simulink model "normalization"  (R2024a)
settings: Solver=VariableStepAuto  StartTime=0.0  StopTime=20  RelTol=1e-3
InitFcn:
  | COL=256;
  | ROW=384;
  | NUM=6;
  | K_COL=COL;
  | K_ROW=ROW/NUM;
  | PLIO_NUM=3;
  | 
  | mtxA_w = [];
  | for i=0:2
  |     pattern = struct('buffer_dimension', [COL,ROW], 'tiling_dimension', [COL,ROW/PLIO_NUM], 'offset', [0,ROW/PLIO_NUM*i]);
  |     mtxA_w = [mtxA_w, pattern];
  | end
  | 
  | mtxA_r = [];
  | for i=0:5
  |     pattern = struct('buffer_dimension', [COL,ROW], 'tiling_dimension', [K_COL,K_ROW], 'offset', [0,K_ROW*i]);
  |     mtxA_r = [mtxA_r, pattern];
  | end
  | 
  | mtxB_w = [];
  | for i=0:5
  |     pattern = struct('buffer_dimension', [COL,ROW], 'tiling_dimension', [K_COL,K_ROW], 'offset', [0,K_ROW*i]);
  |     mtxB_w = [mtxB_w, pattern];
  | end
  | 
  | mtxB_r = [];
  | for i=0:2
  |     pattern = struct('buffer_dimension', [COL,ROW], 'tiling_dimension', [COL,ROW/PLIO_NUM], 'offset', [0,ROW/PLIO_NUM*i]);
  |     mtxB_r = [mtxB_r, pattern];
  | end
  | 
  | inMat = randn(ROW,COL,'single')*2^14;
  | inMatNormalized= (inMat-mean(inMat,'all'))/std(inMat,1,'all');
undefined symbols (not defined in the file or in its folder): aie, AIE, mean_dev_norm_first, mean_dev_norm_last, mean_dev_norm_middle, ML, S, vsvh1760, xcve2802
libraries: aieBasic x14, aieUtilities x10, dspstat3 x2, vmcUtilities x1
settings Model: Creator=robg  LastModifiedBy=sdegala
settings DataIOCC: ReturnWorkspaceOutputs=off
settings SFSimCC: SimTargetLang=C++
settings RTWCC: GPUComputeCapability=3.5

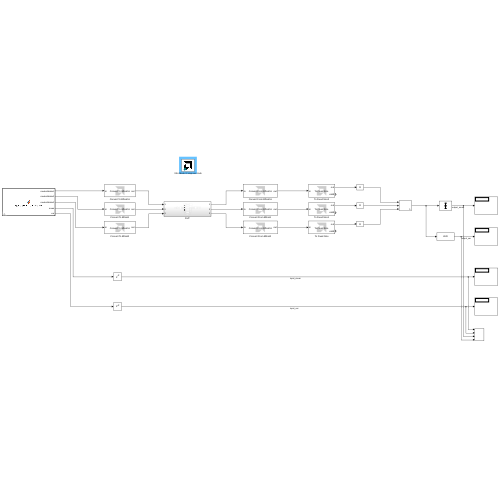
[thumbnail: Simulink's stored preview of the top-level diagram]
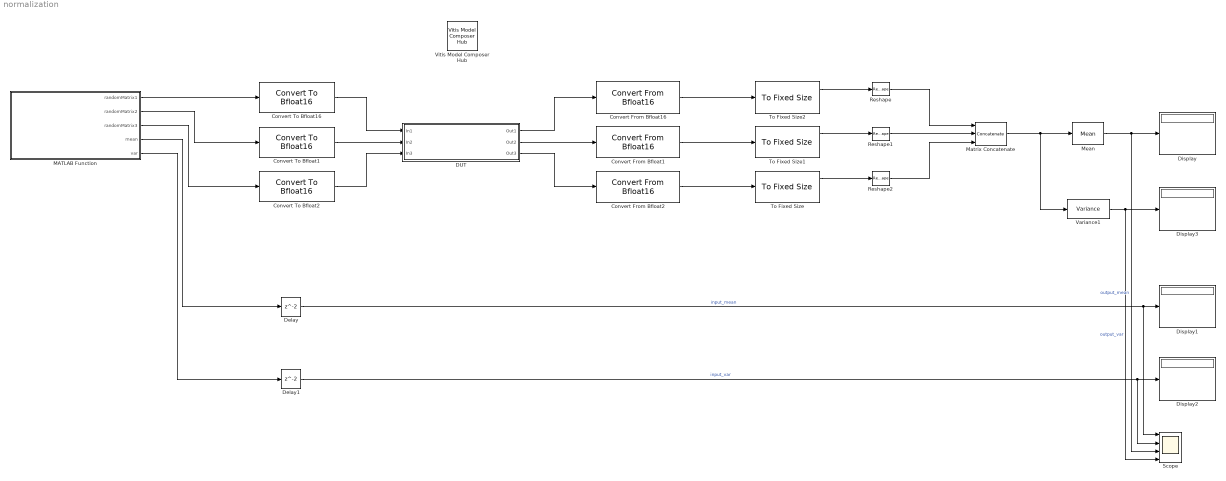
== system normalization ==
  Convert From Bfloat1 : aieUtilities/Convert From Bfloat16  OutputDataType=single
  Convert From Bfloat16 : aieUtilities/Convert From Bfloat16  OutputDataType=single
  Convert From Bfloat2 : aieUtilities/Convert From Bfloat16  OutputDataType=single
  Convert To Bfloat1 : aieUtilities/Convert To Bfloat16
  Convert To Bfloat16 : aieUtilities/Convert To Bfloat16
  Convert To Bfloat2 : aieUtilities/Convert To Bfloat16
  DUT : Subsystem
  Delay : Delay
  Delay1 : Delay
  Display{,1..3} (4 alike) : Display
  MATLAB Function : MATLAB Function  TreatAsAtomicUnit=on  mask{numRows=ROW, numCols=COL}
      mask prompts: numRows "Number of Rows"; numCols "Number of  Columns"
  Matrix Concatenate : Concatenate  NumInputs=3  Mode=Multidimensional array
  Mean : dspstat3/Mean  run=off  InputProcessing=Columns as channels (frame based)  reset_popup=None  directionMode=Entire input  dimension=1  roiEnable=off  roiType=Rectangles  roiPortion=Entire ROI  roiOutput=Individual statistics for each ROI  roiFlag=off  roundingMode=Floor  overflowMode=off  outputDataTypeStr=Inherit: Same as accumulator  outputMin=[]  outputMax=[]  outputLastDataTypeStr=Inherit: Same as accumulator
  Reshape : Reshape  OutputDimensionality=Customize  OutputDimensions=[ROW/PLIO_NUM,COL]
  Reshape1 : Reshape  OutputDimensionality=Customize  OutputDimensions=[ROW/PLIO_NUM,COL]
  Reshape2 : Reshape  OutputDimensionality=Customize  OutputDimensions=[ROW/PLIO_NUM,COL]
  Scope : Scope  NumInputPorts=4
  To Fixed Size : aieUtilities/To Fixed Size  Mode=Produce a valid output signal  OutputSize=Inherit: Same as input  CopyMethod=Buffer samples to form output  HasStatusOutput=on
  To Fixed Size1 : aieUtilities/To Fixed Size  Mode=Produce a valid output signal  OutputSize=Inherit: Same as input  CopyMethod=Buffer samples to form output  HasStatusOutput=on
  To Fixed Size2 : aieUtilities/To Fixed Size  Mode=Produce a valid output signal  OutputSize=Inherit: Same as input  CopyMethod=Buffer samples to form output  HasStatusOutput=on
  Variance1 : dspstat3/Variance  run=off  InputProcessing=Columns as channels (frame based)  reset_popup=None  directionMode=Entire input  dimension=1  roiEnable=off  roiType=Rectangles  roiPortion=Entire ROI  roiOutput=Individual statistics for each ROI  roiFlag=off  roundingMode=Floor  overflowMode=off
  Vitis Model Composer Hub : vmcUtilities/Vitis Model Composer Hub  Tag=genX  CodeGeneration=off  SubsystemName=DUT  BlockHierPath=normalization/DUT  CompilationType=HWCompilation  SubsystemType=AIENode  ExportTypeV2=Graph Code  AIEArrayConfig=Use entire AIE array  StartColumn=1  NumberOfColumns=1  TargetDirectory=./code  exportDesign=on  analyzeDesign=off  validateDesignOnHw=off  ExportType=HW Code  IpVendor=xilinx.com  IpLibrary=hls  IpVersion=1.0  IpHWLanguage=Verilog  AieCompilerOptions={}  AieSimulatorOptions={}  CreateTestbench=off  TestbenchStackSize=10  RunRtlSim=off  RunCSim=off  RunAieSim=on  AieSimTimeout=50000  RunAieSimProfiling=off  LaunchVitisAnalyzer=off  PlotOutput=off  RunX86Sim=off  X86SimTimeout=10  GenHwImage=off  GenLibadfXo=off  GenHwValidationCode=off  PlatformType=Not Specified  HwSystemType=Baremetal  HwValidationTarget=hw  ProjDevice=xcve2802-vsvh1760-2MP-e-S  ProjDevicePart=xcve2802-vsvh1760-2MP-e-S  AIEType=AIE-ML  SamplePeriod=-1  ClockFrequency=200  DataPathParallelism=1  xilinxfamily=versalaiedge  part=xcve2802  speed=-2MP-e-S  package=vsvh1760  directory=./netlist  testbench=off  incr_netlist=off  synthesis_tool=Vivado  clock_wrapper=Clock Enables  dbl_ovrd=According to Block Masks  dcm_input_clock_period=10  sysclk_period=10  simulink_period=1  eval_field=0  IPInfoJsonString="{\"DUTSubsystemName\":\"DUT\",\"AIESubsystem\":{\"SubsystemName\":\"DUT\",\"TargetDirectory\":\"./code\",\"AIEArrayConfig\":\"Use entire AIE array\",\"StartColumn\":\"0\",\"NumberOfColumns\":\"1\"},\"SubsystemTag\":\"AIENode\"}"  LogFileName=/proj/xhdhdstaff5/sdegala/Head1/HEAD/VMC_2025_2_July/Examples/AIENGINE/Normalization/code/model_composer.log  NThreads=4  IPConfigFile=/tmp/vmctmp-6835010160091439353/normalization_ipconfig.json
  wires:
  DUT/1(Out1) -> Convert From Bfloat16/1
  DUT/2(Out2) -> Convert From Bfloat1/1
  DUT/3(Out3) -> Convert From Bfloat2/1
  Convert From Bfloat16/1 -> To Fixed Size2/1
  Convert From Bfloat1/1 -> To Fixed Size1/1
  Convert From Bfloat2/1 -> To Fixed Size/1
  To Fixed Size2/1 -> Reshape/1
  To Fixed Size1/1 -> Reshape1/1
  To Fixed Size/1 -> Reshape2/1
  Reshape/1 -> Matrix Concatenate/1
  Reshape1/1 -> Matrix Concatenate/2
  Reshape2/1 -> Matrix Concatenate/3
  Matrix Concatenate/1 -> Variance1/1, Mean/1
  Mean/1 -> Scope/3, Display/1  "output_mean"
  MATLAB Function/5(var) -> Delay1/1
  Variance1/1 -> Scope/4, Display3/1  "output_var"
  MATLAB Function/4(mean) -> Delay/1
  MATLAB Function/1(randomMatrix1) -> Convert To Bfloat16/1
  MATLAB Function/2(randomMatrix2) -> Convert To Bfloat1/1
  MATLAB Function/3(randomMatrix3) -> Convert To Bfloat2/1
  Convert To Bfloat16/1 -> DUT/1(In1)
  Convert To Bfloat1/1 -> DUT/2(In2)
  Convert To Bfloat2/1 -> DUT/3(In3)
  Delay/1 -> Scope/1, Display1/1  "input_mean"
  Delay1/1 -> Scope/2, Display2/1  "input_var"

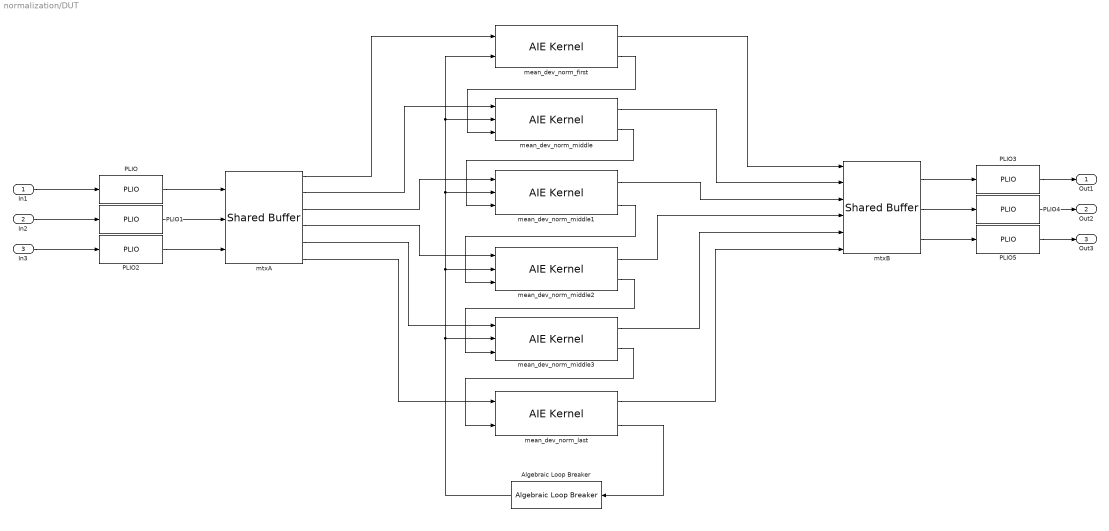
== system normalization/DUT ==
  In1 : Inport
  In2 : Inport  Port=2
  In3 : Inport  Port=3
  Algebraic Loop Breaker : aieUtilities/Algebraic Loop Breaker
  PLIO{,1..5} (6 alike) : aieBasic/PLIO  PlioWidth=128  PlioFreqSpec=off  PlioFreq=250  ColLocation=0  channel=0  blockJsonConstraints=[]  deprecateConstraints=0
  mean_dev_norm_first : aieBasic/AIE Kernel  KernelAllAttrs=|  PortNames={'data'; 'mean_dev'; 'out'; 'partial_out'}  PortSerializedTypes={'{Q2{R{Tadf::input_buffer{1{t{Sbfloat16}}}}}}'; '{Q2{P{Tinput_stream{1{t{Sbfloat16}}}}}}'; '{Q2{R{Tadf::output_buffer{1{t{Sbfloat16}}}}}}'; '{Q2{P{Toutput_cascade{2{t{Saccfloat}}{t{Bv}}}}}}'}  PortWindowSizes={1.600000000000000000e+01, 0.000000000000000000e+00, 1.600000000000000000e+01, 0.000000000000000000e+00}  PortWindowMargins={0.000000000000000000e+00, 0.000000000000000000e+00, 0.000000000000000000e+00, 0.000000000000000000e+00}  PortSynchronicities={'sync', 'auto', 'sync', 'auto'}  PortSignalSizes={0.000000000000000000e+00; 0.000000000000000000e+00; 0.000000000000000000e+00; 3.200000000000000000e+01}  FunctionTemplateSpecKind=implicit  FunctionTemplateParamNames={'COL'; 'ROW'}  FunctionTemplateParamKinds={'nontype'; 'nontype'}  FunctionTemplateParamTypes={'int'; 'int'}  FunctionTemplateParamValues={'0', '0'}  FunctionIndex=1  FunctionTabVisible=on  FunctionTemplateParamsVisible=on  FunctionDeclTypeOptions=|  FunctionDecl=|  FunctionTemplateParams={ 'COL', 'int', 'K_COL'; 'ROW', 'int', 'K_ROW' }  FunctionTemplateParamsEnables={'off', 'off', 'on';'off', 'off', 'on'}  PortAttrs={ 'input', 'data', 'adf::input_buffer< bfloat16 > & restrict', 'K_COL*K_ROW', '0', 'sync', ''; 'input', 'mean_dev', 'input_stream< bfloat16 > * restrict', '', '', '', ''; 'output', 'out', 'adf::output_buffer< bfloat16 > & restrict', 'K_COL*K_ROW', '', 'sync', ''; 'output', 'partial_out', 'output_cascade< accfloat, void > * restrict', '', '', '', '32' }  PortAttrsEnables={'off', 'off', 'off', 'on', 'off', 'off', 'off';'off', 'off', 'off', 'off', 'off', 'off', 'off';'off', 'off', 'off', 'on', 'off', 'off', 'off';'off', 'off', 'off', 'off', 'off', 'off', 'on'}  SampleTime=-1  KernelHeaderFile=aie/kernels.h  KernelFunction=mean_dev_norm_first  KernelSourceFile=aie/mean_dev_norm_first.cc  KernelSearchPaths={}  PreProcOptions={}  blockJsonConstraints=[]
      KernelAllAttrs=|
      | s[12;12;9;9;19;14;21;23;21;23;24;21;15;17;12;24;26;26;26;27;28;9;21;23;23;23;24;25;14;19;19;29]@FunctionNameDeclFileNamePortNamesPortTypesPortSerializedTypesPortDirectionsPortWindowSizeEnablesPortWindowMarginEnablesPortBufferSizeEnablesPortBufferMarginEnablesPortSynchronicityEnablesPortSignalSizeEnablesPortBufferSizesPortBufferMarginsFunctionDeclFunctionTemplateSpecKindFunctionTemplateParamNamesFunctionTemplateParamKindsFunctionTemplateParamTypesFunctionTemplateParamValuesFunctionTemplateParamEnablesClassDeclClassTemplateSpecKindClassTemplateParamNamesClassTemplateParamKindsClassTemplateParamTypesClassTemplateParamValuesClassTemplateParamEnablesClassCtorDeclsClassCtorParamNamesClassCtorParamTypesClassCtorParamSerializedTypes[1 1]@C[32 1]@t19@mean_dev_norm_firstt19@../../aie/kernels.hC[4 1]@t4@datat8@mean_devt3@outt11@partial_outC[4 1]@t40@adf::input_buffer< bfloat16 > & restrictt35@input_stream< bfloat16 > * restrictt41@adf::output_buffer< bfloat16 > & restrictt43@output_cascade< accfloat, void > * restrictC[4 1]@t44@{Q2{R{Tadf::input_buffer{1{t{Sbfloat16}}}}}}t39@{Q2{P{Tinput_stream{1{t{Sbfloat16}}}}}}t45@{Q2{R{Tadf::output_buffer{1{t{Sbfloat16}}}}}}t48@{Q2{P{Toutput_cascade{2{t{Saccfloat}}{t{Bv}}}}}}C[4 1]@t5@inputt5@inputt6@outputt6@outputC[4 1]@l1@l0@l1@l0@C[4 1]@l1@l0@l0@l0@C[4 1]@l1@l0@l1@l0@C[4 1]@l0@l0@l0@l0@C[4 1]@l1@l0@l1@l0@C[4 1]@l0@l0@l0@l1@C[4 1]@nnnnC[4 1]@nnnnt252@template < int COL, int ROW > 
      | void mean_dev_norm_first(adf::input_buffer< bfloat16 > & restrict data, input_stream< bfloat16 > * restrict mean_dev, adf::output_buffer< bfloat16 > & restrict out, output_cascade< accfloat, void > * restrict partial_out)t8@implicitC[2 1]@t3@COLt3@ROWC[2 1]@t7@nontypet7@nontypeC[2 1]@t3@intt3@intC[2 1]@nnC[2 1]@l1@l1@nne[0 1]@e[0 1]@e[0 1]@e[0 1]@e[0 1]@e[0 1]@e[0 1]@e[0 1]@e[0 1]@
      FunctionDeclTypeOptions=|
      | C[1 1]@t254@template < int COL, int ROW > 
      | void mean_dev_norm_first(adf::input_buffer< bfloat16 > && restrict data, input_stream< bfloat16 > * restrict mean_dev, adf::output_buffer< bfloat16 > && restrict out, output_cascade< accfloat, void > * restrict partial_out)
      FunctionDecl=|
      | template < int COL, int ROW > 
      | void mean_dev_norm_first(adf::input_buffer< bfloat16 > && restrict data, input_stream< bfloat16 > * restrict mean_dev, adf::output_buffer< bfloat16 > && restrict out, output_cascade< accfloat, void > * restrict partial_out)
  mean_dev_norm_last : aieBasic/AIE Kernel  KernelAllAttrs=|  PortNames={'data'; 'partial_in'; 'out'; 'mean_dev_out'}  PortSerializedTypes={'{Q2{R{Tadf::input_buffer{1{t{Sbfloat16}}}}}}'; '{Q2{P{Tinput_cascade{2{t{Saccfloat}}{t{Bv}}}}}}'; '{Q2{R{Tadf::output_buffer{1{t{Sbfloat16}}}}}}'; '{Q2{P{Toutput_stream{1{t{Sbfloat16}}}}}}'}  PortWindowSizes={1.600000000000000000e+01, 0.000000000000000000e+00, 1.600000000000000000e+01, 0.000000000000000000e+00}  PortWindowMargins={0.000000000000000000e+00, 0.000000000000000000e+00, 0.000000000000000000e+00, 0.000000000000000000e+00}  PortSynchronicities={'sync', 'auto', 'sync', 'auto'}  PortSignalSizes={0.000000000000000000e+00; 0.000000000000000000e+00; 0.000000000000000000e+00; 2.000000000000000000e+00}  FunctionTemplateSpecKind=implicit  FunctionTemplateParamNames={'COL'; 'ROW'; 'NUM'}  FunctionTemplateParamKinds={'nontype'; 'nontype'; 'nontype'}  FunctionTemplateParamTypes={'int'; 'int'; 'int'}  FunctionTemplateParamValues={'0', '0', '0'}  FunctionIndex=1  FunctionTabVisible=on  FunctionTemplateParamsVisible=on  FunctionDeclTypeOptions=|  FunctionDecl=|  FunctionTemplateParams={ 'COL', 'int', 'K_COL'; 'ROW', 'int', 'K_ROW'; 'NUM', 'int', 'NUM' }  FunctionTemplateParamsEnables={'off', 'off', 'on';'off', 'off', 'on';'off', 'off', 'on'}  PortAttrs={ 'input', 'data', 'adf::input_buffer< bfloat16 > & restrict', 'K_COL*K_ROW', '0', 'sync', ''; 'input', 'partial_in', 'input_cascade< accfloat, void > * restrict', '', '', '', ''; 'output', 'out', 'adf::output_buffer< bfloat16 > & restrict', 'K_COL*K_ROW', '', 'sync', ''; 'output', 'mean_dev_out', 'output_stream< bfloat16 > * restrict', '', '', '', '2' }  PortAttrsEnables={'off', 'off', 'off', 'on', 'off', 'off', 'off';'off', 'off', 'off', 'off', 'off', 'off', 'off';'off', 'off', 'off', 'on', 'off', 'off', 'off';'off', 'off', 'off', 'off', 'off', 'off', 'on'}  SampleTime=-1  KernelHeaderFile=aie/kernels.h  KernelFunction=mean_dev_norm_last  KernelSourceFile=aie/mean_dev_norm_last.cc  KernelSearchPaths={}  PreProcOptions={}  blockJsonConstraints=[]
      KernelAllAttrs=|
      | s[12;12;9;9;19;14;21;23;21;23;24;21;15;17;12;24;26;26;26;27;28;9;21;23;23;23;24;25;14;19;19;29]@FunctionNameDeclFileNamePortNamesPortTypesPortSerializedTypesPortDirectionsPortWindowSizeEnablesPortWindowMarginEnablesPortBufferSizeEnablesPortBufferMarginEnablesPortSynchronicityEnablesPortSignalSizeEnablesPortBufferSizesPortBufferMarginsFunctionDeclFunctionTemplateSpecKindFunctionTemplateParamNamesFunctionTemplateParamKindsFunctionTemplateParamTypesFunctionTemplateParamValuesFunctionTemplateParamEnablesClassDeclClassTemplateSpecKindClassTemplateParamNamesClassTemplateParamKindsClassTemplateParamTypesClassTemplateParamValuesClassTemplateParamEnablesClassCtorDeclsClassCtorParamNamesClassCtorParamTypesClassCtorParamSerializedTypes[1 1]@C[32 1]@t18@mean_dev_norm_lastt19@../../aie/kernels.hC[4 1]@t4@datat10@partial_int3@outt12@mean_dev_outC[4 1]@t40@adf::input_buffer< bfloat16 > & restrictt42@input_cascade< accfloat, void > * restrictt41@adf::output_buffer< bfloat16 > & restrictt36@output_stream< bfloat16 > * restrictC[4 1]@t44@{Q2{R{Tadf::input_buffer{1{t{Sbfloat16}}}}}}t47@{Q2{P{Tinput_cascade{2{t{Saccfloat}}{t{Bv}}}}}}t45@{Q2{R{Tadf::output_buffer{1{t{Sbfloat16}}}}}}t40@{Q2{P{Toutput_stream{1{t{Sbfloat16}}}}}}C[4 1]@t5@inputt5@inputt6@outputt6@outputC[4 1]@l1@l0@l1@l0@C[4 1]@l1@l0@l0@l0@C[4 1]@l1@l0@l1@l0@C[4 1]@l0@l0@l0@l0@C[4 1]@l1@l0@l1@l0@C[4 1]@l0@l0@l0@l1@C[4 1]@nnnnC[4 1]@nnnnt263@template < int COL, int ROW, int NUM > 
      | void mean_dev_norm_last(adf::input_buffer< bfloat16 > & restrict data, input_cascade< accfloat, void > * restrict partial_in, adf::output_buffer< bfloat16 > & restrict out, output_stream< bfloat16 > * restrict mean_dev_out)t8@implicitC[3 1]@t3@COLt3@ROWt3@NUMC[3 1]@t7@nontypet7@nontypet7@nontypeC[3 1]@t3@intt3@intt3@intC[3 1]@nnnC[3 1]@l1@l1@l1@nne[0 1]@e[0 1]@e[0 1]@e[0 1]@e[0 1]@e[0 1]@e[0 1]@e[0 1]@e[0 1]@
      FunctionDeclTypeOptions=|
      | C[1 1]@t265@template < int COL, int ROW, int NUM > 
      | void mean_dev_norm_last(adf::input_buffer< bfloat16 > && restrict data, input_cascade< accfloat, void > * restrict partial_in, adf::output_buffer< bfloat16 > && restrict out, output_stream< bfloat16 > * restrict mean_dev_out)
      FunctionDecl=|
      | template < int COL, int ROW, int NUM > 
      | void mean_dev_norm_last(adf::input_buffer< bfloat16 > && restrict data, input_cascade< accfloat, void > * restrict partial_in, adf::output_buffer< bfloat16 > && restrict out, output_stream< bfloat16 > * restrict mean_dev_out)
  mean_dev_norm_middle : aieBasic/AIE Kernel  KernelAllAttrs=|  PortNames={'data'; 'mean_dev'; 'partial_in'; 'out'; 'partial_out'}  PortSerializedTypes={'{Q2{R{Tadf::input_buffer{1{t{Sbfloat16}}}}}}'; '{Q2{P{Tinput_stream{1{t{Sbfloat16}}}}}}'; '{Q2{P{Tinput_cascade{2{t{Saccfloat}}{t{Bv}}}}}}'; '{Q2{R{Tadf::output_buffer{1{t{Sbfloat16}}}}}}'; '{Q2{P{Toutput_cascade{2{t{Saccfloat}}{t{Bv}}}}}}'}  PortWindowSizes={1.600000000000000000e+01, 0.000000000000000000e+00, 0.000000000000000000e+00, 1.600000000000000000e+01, 0.000000000000000000e+00}  PortWindowMargins={0.000000000000000000e+00, 0.000000000000000000e+00, 0.000000000000000000e+00, 0.000000000000000000e+00, 0.000000000000000000e+00}  PortSynchronicities={'sync', 'auto', 'auto', 'sync', 'auto'}  PortSignalSizes={0.000000000000000000e+00; 0.000000000000000000e+00; 0.000000000000000000e+00; 0.000000000000000000e+00; 3.200000000000000000e+01}  FunctionTemplateSpecKind=implicit  FunctionTemplateParamNames={'COL'; 'ROW'}  FunctionTemplateParamKinds={'nontype'; 'nontype'}  FunctionTemplateParamTypes={'int'; 'int'}  FunctionTemplateParamValues={'0', '0'}  FunctionIndex=1  FunctionTabVisible=on  FunctionTemplateParamsVisible=on  FunctionDeclTypeOptions=|  FunctionDecl=|  FunctionTemplateParams={ 'COL', 'int', 'K_COL'; 'ROW', 'int', 'K_ROW' }  FunctionTemplateParamsEnables={'off', 'off', 'on';'off', 'off', 'on'}  PortAttrs={ 'input', 'data', 'adf::input_buffer< bfloat16 > & restrict', 'K_COL*K_ROW', '0', 'sync', ''; 'input', 'mean_dev', 'input_stream< bfloat16 > * restrict', '', '', '', ''; 'input', 'partial_in', 'input_cascade< accfloat, void > * restrict', '', '', '', ''; 'output', 'out', 'adf::output_buffer< bfloat16 > & restrict', 'K_COL*K_ROW', '', 'sync', ''; 'output', 'partial_out', 'output_cascade< accfloat, void > * restrict', '', '', '', '32' }  PortAttrsEnables={'off', 'off', 'off', 'on', 'off', 'off', 'off';'off', 'off', 'off', 'off', 'off', 'off', 'off';'off', 'off', 'off', 'off', 'off', 'off', 'off';'off', 'off', 'off', 'on', 'off', 'off', 'off';'off', 'off', 'off', 'off', 'off', 'off', 'on'}  SampleTime=-1  KernelHeaderFile=aie/kernels.h  KernelFunction=mean_dev_norm_middle  KernelSourceFile=aie/mean_dev_norm_middle.cc  KernelSearchPaths={}  PreProcOptions={}  blockJsonConstraints=[]
      KernelAllAttrs=|
      | s[12;12;9;9;19;14;21;23;21;23;24;21;15;17;12;24;26;26;26;27;28;9;21;23;23;23;24;25;14;19;19;29]@FunctionNameDeclFileNamePortNamesPortTypesPortSerializedTypesPortDirectionsPortWindowSizeEnablesPortWindowMarginEnablesPortBufferSizeEnablesPortBufferMarginEnablesPortSynchronicityEnablesPortSignalSizeEnablesPortBufferSizesPortBufferMarginsFunctionDeclFunctionTemplateSpecKindFunctionTemplateParamNamesFunctionTemplateParamKindsFunctionTemplateParamTypesFunctionTemplateParamValuesFunctionTemplateParamEnablesClassDeclClassTemplateSpecKindClassTemplateParamNamesClassTemplateParamKindsClassTemplateParamTypesClassTemplateParamValuesClassTemplateParamEnablesClassCtorDeclsClassCtorParamNamesClassCtorParamTypesClassCtorParamSerializedTypes[1 1]@C[32 1]@t20@mean_dev_norm_middlet19@../../aie/kernels.hC[5 1]@t4@datat8@mean_devt10@partial_int3@outt11@partial_outC[5 1]@t40@adf::input_buffer< bfloat16 > & restrictt35@input_stream< bfloat16 > * restrictt42@input_cascade< accfloat, void > * restrictt41@adf::output_buffer< bfloat16 > & restrictt43@output_cascade< accfloat, void > * restrictC[5 1]@t44@{Q2{R{Tadf::input_buffer{1{t{Sbfloat16}}}}}}t39@{Q2{P{Tinput_stream{1{t{Sbfloat16}}}}}}t47@{Q2{P{Tinput_cascade{2{t{Saccfloat}}{t{Bv}}}}}}t45@{Q2{R{Tadf::output_buffer{1{t{Sbfloat16}}}}}}t48@{Q2{P{Toutput_cascade{2{t{Saccfloat}}{t{Bv}}}}}}C[5 1]@t5@inputt5@inputt5@inputt6@outputt6@outputC[5 1]@l1@l0@l0@l1@l0@C[5 1]@l1@l0@l0@l0@l0@C[5 1]@l1@l0@l0@l1@l0@C[5 1]@l0@l0@l0@l0@l0@C[5 1]@l1@l0@l0@l1@l0@C[5 1]@l0@l0@l0@l0@l1@C[5 1]@nnnnnC[5 1]@nnnnnt308@template < int COL, int ROW > 
      | void mean_dev_norm_middle(adf::input_buffer< bfloat16 > & restrict data, input_stream< bfloat16 > * restrict mean_dev, input_cascade< accfloat, void > * restrict partial_in, adf::output_buffer< bfloat16 > & restrict out, output_cascade< accfloat, void > * restrict partial_out)t8@implicitC[2 1]@t3@COLt3@ROWC[2 1]@t7@nontypet7@nontypeC[2 1]@t3@intt3@intC[2 1]@nnC[2 1]@l1@l1@nne[0 1]@e[0 1]@e[0 1]@e[0 1]@e[0 1]@e[0 1]@e[0 1]@e[0 1]@e[0 1]@
      FunctionDeclTypeOptions=|
      | C[1 1]@t310@template < int COL, int ROW > 
      | void mean_dev_norm_middle(adf::input_buffer< bfloat16 > && restrict data, input_stream< bfloat16 > * restrict mean_dev, input_cascade< accfloat, void > * restrict partial_in, adf::output_buffer< bfloat16 > && restrict out, output_cascade< accfloat, void > * restrict partial_out)
      FunctionDecl=|
      | template < int COL, int ROW > 
      | void mean_dev_norm_middle(adf::input_buffer< bfloat16 > && restrict data, input_stream< bfloat16 > * restrict mean_dev, input_cascade< accfloat, void > * restrict partial_in, adf::output_buffer< bfloat16 > && restrict out, output_cascade< accfloat, void > * restrict partial_out)
  mean_dev_norm_middle1 : aieBasic/AIE Kernel  KernelAllAttrs=|  PortNames={'data'; 'mean_dev'; 'partial_in'; 'out'; 'partial_out'}  PortSerializedTypes={'{Q2{R{Tadf::input_buffer{1{t{Sbfloat16}}}}}}'; '{Q2{P{Tinput_stream{1{t{Sbfloat16}}}}}}'; '{Q2{P{Tinput_cascade{2{t{Saccfloat}}{t{Bv}}}}}}'; '{Q2{R{Tadf::output_buffer{1{t{Sbfloat16}}}}}}'; '{Q2{P{Toutput_cascade{2{t{Saccfloat}}{t{Bv}}}}}}'}  PortWindowSizes={1.600000000000000000e+01, 0.000000000000000000e+00, 0.000000000000000000e+00, 1.600000000000000000e+01, 0.000000000000000000e+00}  PortWindowMargins={0.000000000000000000e+00, 0.000000000000000000e+00, 0.000000000000000000e+00, 0.000000000000000000e+00, 0.000000000000000000e+00}  PortSynchronicities={'sync', 'auto', 'auto', 'sync', 'auto'}  PortSignalSizes={0.000000000000000000e+00; 0.000000000000000000e+00; 0.000000000000000000e+00; 0.000000000000000000e+00; 3.200000000000000000e+01}  FunctionTemplateSpecKind=implicit  FunctionTemplateParamNames={'COL'; 'ROW'}  FunctionTemplateParamKinds={'nontype'; 'nontype'}  FunctionTemplateParamTypes={'int'; 'int'}  FunctionTemplateParamValues={'0', '0'}  FunctionIndex=1  FunctionTabVisible=on  FunctionTemplateParamsVisible=on  FunctionDeclTypeOptions=|  FunctionDecl=|  FunctionTemplateParams={ 'COL', 'int', 'K_COL'; 'ROW', 'int', 'K_ROW' }  FunctionTemplateParamsEnables={'off', 'off', 'on';'off', 'off', 'on'}  PortAttrs={ 'input', 'data', 'adf::input_buffer< bfloat16 > & restrict', 'K_COL*K_ROW', '0', 'sync', ''; 'input', 'mean_dev', 'input_stream< bfloat16 > * restrict', '', '', '', ''; 'input', 'partial_in', 'input_cascade< accfloat, void > * restrict', '', '', '', ''; 'output', 'out', 'adf::output_buffer< bfloat16 > & restrict', 'K_COL*K_ROW', '', 'sync', ''; 'output', 'partial_out', 'output_cascade< accfloat, void > * restrict', '', '', '', '32' }  PortAttrsEnables={'off', 'off', 'off', 'on', 'off', 'off', 'off';'off', 'off', 'off', 'off', 'off', 'off', 'off';'off', 'off', 'off', 'off', 'off', 'off', 'off';'off', 'off', 'off', 'on', 'off', 'off', 'off';'off', 'off', 'off', 'off', 'off', 'off', 'on'}  SampleTime=-1  KernelHeaderFile=aie/kernels.h  KernelFunction=mean_dev_norm_middle  KernelSourceFile=aie/mean_dev_norm_middle.cc  KernelSearchPaths={}  PreProcOptions={}  blockJsonConstraints=[]
      KernelAllAttrs=|
      | s[12;12;9;9;19;14;21;23;21;23;24;21;15;17;12;24;26;26;26;27;28;9;21;23;23;23;24;25;14;19;19;29]@FunctionNameDeclFileNamePortNamesPortTypesPortSerializedTypesPortDirectionsPortWindowSizeEnablesPortWindowMarginEnablesPortBufferSizeEnablesPortBufferMarginEnablesPortSynchronicityEnablesPortSignalSizeEnablesPortBufferSizesPortBufferMarginsFunctionDeclFunctionTemplateSpecKindFunctionTemplateParamNamesFunctionTemplateParamKindsFunctionTemplateParamTypesFunctionTemplateParamValuesFunctionTemplateParamEnablesClassDeclClassTemplateSpecKindClassTemplateParamNamesClassTemplateParamKindsClassTemplateParamTypesClassTemplateParamValuesClassTemplateParamEnablesClassCtorDeclsClassCtorParamNamesClassCtorParamTypesClassCtorParamSerializedTypes[1 1]@C[32 1]@t20@mean_dev_norm_middlet19@../../aie/kernels.hC[5 1]@t4@datat8@mean_devt10@partial_int3@outt11@partial_outC[5 1]@t40@adf::input_buffer< bfloat16 > & restrictt35@input_stream< bfloat16 > * restrictt42@input_cascade< accfloat, void > * restrictt41@adf::output_buffer< bfloat16 > & restrictt43@output_cascade< accfloat, void > * restrictC[5 1]@t44@{Q2{R{Tadf::input_buffer{1{t{Sbfloat16}}}}}}t39@{Q2{P{Tinput_stream{1{t{Sbfloat16}}}}}}t47@{Q2{P{Tinput_cascade{2{t{Saccfloat}}{t{Bv}}}}}}t45@{Q2{R{Tadf::output_buffer{1{t{Sbfloat16}}}}}}t48@{Q2{P{Toutput_cascade{2{t{Saccfloat}}{t{Bv}}}}}}C[5 1]@t5@inputt5@inputt5@inputt6@outputt6@outputC[5 1]@l1@l0@l0@l1@l0@C[5 1]@l1@l0@l0@l0@l0@C[5 1]@l1@l0@l0@l1@l0@C[5 1]@l0@l0@l0@l0@l0@C[5 1]@l1@l0@l0@l1@l0@C[5 1]@l0@l0@l0@l0@l1@C[5 1]@nnnnnC[5 1]@nnnnnt308@template < int COL, int ROW > 
      | void mean_dev_norm_middle(adf::input_buffer< bfloat16 > & restrict data, input_stream< bfloat16 > * restrict mean_dev, input_cascade< accfloat, void > * restrict partial_in, adf::output_buffer< bfloat16 > & restrict out, output_cascade< accfloat, void > * restrict partial_out)t8@implicitC[2 1]@t3@COLt3@ROWC[2 1]@t7@nontypet7@nontypeC[2 1]@t3@intt3@intC[2 1]@nnC[2 1]@l1@l1@nne[0 1]@e[0 1]@e[0 1]@e[0 1]@e[0 1]@e[0 1]@e[0 1]@e[0 1]@e[0 1]@
      FunctionDeclTypeOptions=|
      | C[1 1]@t310@template < int COL, int ROW > 
      | void mean_dev_norm_middle(adf::input_buffer< bfloat16 > && restrict data, input_stream< bfloat16 > * restrict mean_dev, input_cascade< accfloat, void > * restrict partial_in, adf::output_buffer< bfloat16 > && restrict out, output_cascade< accfloat, void > * restrict partial_out)
      FunctionDecl=|
      | template < int COL, int ROW > 
      | void mean_dev_norm_middle(adf::input_buffer< bfloat16 > && restrict data, input_stream< bfloat16 > * restrict mean_dev, input_cascade< accfloat, void > * restrict partial_in, adf::output_buffer< bfloat16 > && restrict out, output_cascade< accfloat, void > * restrict partial_out)
  mean_dev_norm_middle2 : aieBasic/AIE Kernel  KernelAllAttrs=|  PortNames={'data'; 'mean_dev'; 'partial_in'; 'out'; 'partial_out'}  PortSerializedTypes={'{Q2{R{Tadf::input_buffer{1{t{Sbfloat16}}}}}}'; '{Q2{P{Tinput_stream{1{t{Sbfloat16}}}}}}'; '{Q2{P{Tinput_cascade{2{t{Saccfloat}}{t{Bv}}}}}}'; '{Q2{R{Tadf::output_buffer{1{t{Sbfloat16}}}}}}'; '{Q2{P{Toutput_cascade{2{t{Saccfloat}}{t{Bv}}}}}}'}  PortWindowSizes={1.600000000000000000e+01, 0.000000000000000000e+00, 0.000000000000000000e+00, 1.600000000000000000e+01, 0.000000000000000000e+00}  PortWindowMargins={0.000000000000000000e+00, 0.000000000000000000e+00, 0.000000000000000000e+00, 0.000000000000000000e+00, 0.000000000000000000e+00}  PortSynchronicities={'sync', 'auto', 'auto', 'sync', 'auto'}  PortSignalSizes={0.000000000000000000e+00; 0.000000000000000000e+00; 0.000000000000000000e+00; 0.000000000000000000e+00; 3.200000000000000000e+01}  FunctionTemplateSpecKind=implicit  FunctionTemplateParamNames={'COL'; 'ROW'}  FunctionTemplateParamKinds={'nontype'; 'nontype'}  FunctionTemplateParamTypes={'int'; 'int'}  FunctionTemplateParamValues={'0', '0'}  FunctionIndex=1  FunctionTabVisible=on  FunctionTemplateParamsVisible=on  FunctionDeclTypeOptions=|  FunctionDecl=|  FunctionTemplateParams={ 'COL', 'int', 'K_COL'; 'ROW', 'int', 'K_ROW' }  FunctionTemplateParamsEnables={'off', 'off', 'on';'off', 'off', 'on'}  PortAttrs={ 'input', 'data', 'adf::input_buffer< bfloat16 > & restrict', 'K_COL*K_ROW', '0', 'sync', ''; 'input', 'mean_dev', 'input_stream< bfloat16 > * restrict', '', '', '', ''; 'input', 'partial_in', 'input_cascade< accfloat, void > * restrict', '', '', '', ''; 'output', 'out', 'adf::output_buffer< bfloat16 > & restrict', 'K_COL*K_ROW', '', 'sync', ''; 'output', 'partial_out', 'output_cascade< accfloat, void > * restrict', '', '', '', '32' }  PortAttrsEnables={'off', 'off', 'off', 'on', 'off', 'off', 'off';'off', 'off', 'off', 'off', 'off', 'off', 'off';'off', 'off', 'off', 'off', 'off', 'off', 'off';'off', 'off', 'off', 'on', 'off', 'off', 'off';'off', 'off', 'off', 'off', 'off', 'off', 'on'}  SampleTime=-1  KernelHeaderFile=aie/kernels.h  KernelFunction=mean_dev_norm_middle  KernelSourceFile=aie/mean_dev_norm_middle.cc  KernelSearchPaths={}  PreProcOptions={}  blockJsonConstraints=[]
      KernelAllAttrs=|
      | s[12;12;9;9;19;14;21;23;21;23;24;21;15;17;12;24;26;26;26;27;28;9;21;23;23;23;24;25;14;19;19;29]@FunctionNameDeclFileNamePortNamesPortTypesPortSerializedTypesPortDirectionsPortWindowSizeEnablesPortWindowMarginEnablesPortBufferSizeEnablesPortBufferMarginEnablesPortSynchronicityEnablesPortSignalSizeEnablesPortBufferSizesPortBufferMarginsFunctionDeclFunctionTemplateSpecKindFunctionTemplateParamNamesFunctionTemplateParamKindsFunctionTemplateParamTypesFunctionTemplateParamValuesFunctionTemplateParamEnablesClassDeclClassTemplateSpecKindClassTemplateParamNamesClassTemplateParamKindsClassTemplateParamTypesClassTemplateParamValuesClassTemplateParamEnablesClassCtorDeclsClassCtorParamNamesClassCtorParamTypesClassCtorParamSerializedTypes[1 1]@C[32 1]@t20@mean_dev_norm_middlet19@../../aie/kernels.hC[5 1]@t4@datat8@mean_devt10@partial_int3@outt11@partial_outC[5 1]@t40@adf::input_buffer< bfloat16 > & restrictt35@input_stream< bfloat16 > * restrictt42@input_cascade< accfloat, void > * restrictt41@adf::output_buffer< bfloat16 > & restrictt43@output_cascade< accfloat, void > * restrictC[5 1]@t44@{Q2{R{Tadf::input_buffer{1{t{Sbfloat16}}}}}}t39@{Q2{P{Tinput_stream{1{t{Sbfloat16}}}}}}t47@{Q2{P{Tinput_cascade{2{t{Saccfloat}}{t{Bv}}}}}}t45@{Q2{R{Tadf::output_buffer{1{t{Sbfloat16}}}}}}t48@{Q2{P{Toutput_cascade{2{t{Saccfloat}}{t{Bv}}}}}}C[5 1]@t5@inputt5@inputt5@inputt6@outputt6@outputC[5 1]@l1@l0@l0@l1@l0@C[5 1]@l1@l0@l0@l0@l0@C[5 1]@l1@l0@l0@l1@l0@C[5 1]@l0@l0@l0@l0@l0@C[5 1]@l1@l0@l0@l1@l0@C[5 1]@l0@l0@l0@l0@l1@C[5 1]@nnnnnC[5 1]@nnnnnt308@template < int COL, int ROW > 
      | void mean_dev_norm_middle(adf::input_buffer< bfloat16 > & restrict data, input_stream< bfloat16 > * restrict mean_dev, input_cascade< accfloat, void > * restrict partial_in, adf::output_buffer< bfloat16 > & restrict out, output_cascade< accfloat, void > * restrict partial_out)t8@implicitC[2 1]@t3@COLt3@ROWC[2 1]@t7@nontypet7@nontypeC[2 1]@t3@intt3@intC[2 1]@nnC[2 1]@l1@l1@nne[0 1]@e[0 1]@e[0 1]@e[0 1]@e[0 1]@e[0 1]@e[0 1]@e[0 1]@e[0 1]@
      FunctionDeclTypeOptions=|
      | C[1 1]@t310@template < int COL, int ROW > 
      | void mean_dev_norm_middle(adf::input_buffer< bfloat16 > && restrict data, input_stream< bfloat16 > * restrict mean_dev, input_cascade< accfloat, void > * restrict partial_in, adf::output_buffer< bfloat16 > && restrict out, output_cascade< accfloat, void > * restrict partial_out)
      FunctionDecl=|
      | template < int COL, int ROW > 
      | void mean_dev_norm_middle(adf::input_buffer< bfloat16 > && restrict data, input_stream< bfloat16 > * restrict mean_dev, input_cascade< accfloat, void > * restrict partial_in, adf::output_buffer< bfloat16 > && restrict out, output_cascade< accfloat, void > * restrict partial_out)
  mean_dev_norm_middle3 : aieBasic/AIE Kernel  KernelAllAttrs=|  PortNames={'data'; 'mean_dev'; 'partial_in'; 'out'; 'partial_out'}  PortSerializedTypes={'{Q2{R{Tadf::input_buffer{1{t{Sbfloat16}}}}}}'; '{Q2{P{Tinput_stream{1{t{Sbfloat16}}}}}}'; '{Q2{P{Tinput_cascade{2{t{Saccfloat}}{t{Bv}}}}}}'; '{Q2{R{Tadf::output_buffer{1{t{Sbfloat16}}}}}}'; '{Q2{P{Toutput_cascade{2{t{Saccfloat}}{t{Bv}}}}}}'}  PortWindowSizes={1.600000000000000000e+01, 0.000000000000000000e+00, 0.000000000000000000e+00, 1.600000000000000000e+01, 0.000000000000000000e+00}  PortWindowMargins={0.000000000000000000e+00, 0.000000000000000000e+00, 0.000000000000000000e+00, 0.000000000000000000e+00, 0.000000000000000000e+00}  PortSynchronicities={'sync', 'auto', 'auto', 'sync', 'auto'}  PortSignalSizes={0.000000000000000000e+00; 0.000000000000000000e+00; 0.000000000000000000e+00; 0.000000000000000000e+00; 3.200000000000000000e+01}  FunctionTemplateSpecKind=implicit  FunctionTemplateParamNames={'COL'; 'ROW'}  FunctionTemplateParamKinds={'nontype'; 'nontype'}  FunctionTemplateParamTypes={'int'; 'int'}  FunctionTemplateParamValues={'0', '0'}  FunctionIndex=1  FunctionTabVisible=on  FunctionTemplateParamsVisible=on  FunctionDeclTypeOptions=|  FunctionDecl=|  FunctionTemplateParams={ 'COL', 'int', 'K_COL'; 'ROW', 'int', 'K_ROW' }  FunctionTemplateParamsEnables={'off', 'off', 'on';'off', 'off', 'on'}  PortAttrs={ 'input', 'data', 'adf::input_buffer< bfloat16 > & restrict', 'K_COL*K_ROW', '0', 'sync', ''; 'input', 'mean_dev', 'input_stream< bfloat16 > * restrict', '', '', '', ''; 'input', 'partial_in', 'input_cascade< accfloat, void > * restrict', '', '', '', ''; 'output', 'out', 'adf::output_buffer< bfloat16 > & restrict', 'K_COL*K_ROW', '', 'sync', ''; 'output', 'partial_out', 'output_cascade< accfloat, void > * restrict', '', '', '', '32' }  PortAttrsEnables={'off', 'off', 'off', 'on', 'off', 'off', 'off';'off', 'off', 'off', 'off', 'off', 'off', 'off';'off', 'off', 'off', 'off', 'off', 'off', 'off';'off', 'off', 'off', 'on', 'off', 'off', 'off';'off', 'off', 'off', 'off', 'off', 'off', 'on'}  SampleTime=-1  KernelHeaderFile=aie/kernels.h  KernelFunction=mean_dev_norm_middle  KernelSourceFile=aie/mean_dev_norm_middle.cc  KernelSearchPaths={}  PreProcOptions={}  blockJsonConstraints=[]
      KernelAllAttrs=|
      | s[12;12;9;9;19;14;21;23;21;23;24;21;15;17;12;24;26;26;26;27;28;9;21;23;23;23;24;25;14;19;19;29]@FunctionNameDeclFileNamePortNamesPortTypesPortSerializedTypesPortDirectionsPortWindowSizeEnablesPortWindowMarginEnablesPortBufferSizeEnablesPortBufferMarginEnablesPortSynchronicityEnablesPortSignalSizeEnablesPortBufferSizesPortBufferMarginsFunctionDeclFunctionTemplateSpecKindFunctionTemplateParamNamesFunctionTemplateParamKindsFunctionTemplateParamTypesFunctionTemplateParamValuesFunctionTemplateParamEnablesClassDeclClassTemplateSpecKindClassTemplateParamNamesClassTemplateParamKindsClassTemplateParamTypesClassTemplateParamValuesClassTemplateParamEnablesClassCtorDeclsClassCtorParamNamesClassCtorParamTypesClassCtorParamSerializedTypes[1 1]@C[32 1]@t20@mean_dev_norm_middlet19@../../aie/kernels.hC[5 1]@t4@datat8@mean_devt10@partial_int3@outt11@partial_outC[5 1]@t40@adf::input_buffer< bfloat16 > & restrictt35@input_stream< bfloat16 > * restrictt42@input_cascade< accfloat, void > * restrictt41@adf::output_buffer< bfloat16 > & restrictt43@output_cascade< accfloat, void > * restrictC[5 1]@t44@{Q2{R{Tadf::input_buffer{1{t{Sbfloat16}}}}}}t39@{Q2{P{Tinput_stream{1{t{Sbfloat16}}}}}}t47@{Q2{P{Tinput_cascade{2{t{Saccfloat}}{t{Bv}}}}}}t45@{Q2{R{Tadf::output_buffer{1{t{Sbfloat16}}}}}}t48@{Q2{P{Toutput_cascade{2{t{Saccfloat}}{t{Bv}}}}}}C[5 1]@t5@inputt5@inputt5@inputt6@outputt6@outputC[5 1]@l1@l0@l0@l1@l0@C[5 1]@l1@l0@l0@l0@l0@C[5 1]@l1@l0@l0@l1@l0@C[5 1]@l0@l0@l0@l0@l0@C[5 1]@l1@l0@l0@l1@l0@C[5 1]@l0@l0@l0@l0@l1@C[5 1]@nnnnnC[5 1]@nnnnnt308@template < int COL, int ROW > 
      | void mean_dev_norm_middle(adf::input_buffer< bfloat16 > & restrict data, input_stream< bfloat16 > * restrict mean_dev, input_cascade< accfloat, void > * restrict partial_in, adf::output_buffer< bfloat16 > & restrict out, output_cascade< accfloat, void > * restrict partial_out)t8@implicitC[2 1]@t3@COLt3@ROWC[2 1]@t7@nontypet7@nontypeC[2 1]@t3@intt3@intC[2 1]@nnC[2 1]@l1@l1@nne[0 1]@e[0 1]@e[0 1]@e[0 1]@e[0 1]@e[0 1]@e[0 1]@e[0 1]@e[0 1]@
      FunctionDeclTypeOptions=|
      | C[1 1]@t310@template < int COL, int ROW > 
      | void mean_dev_norm_middle(adf::input_buffer< bfloat16 > && restrict data, input_stream< bfloat16 > * restrict mean_dev, input_cascade< accfloat, void > * restrict partial_in, adf::output_buffer< bfloat16 > && restrict out, output_cascade< accfloat, void > * restrict partial_out)
      FunctionDecl=|
      | template < int COL, int ROW > 
      | void mean_dev_norm_middle(adf::input_buffer< bfloat16 > && restrict data, input_stream< bfloat16 > * restrict mean_dev, input_cascade< accfloat, void > * restrict partial_in, adf::output_buffer< bfloat16 > && restrict out, output_cascade< accfloat, void > * restrict partial_out)
  mtxA : aieBasic/Shared Buffer  DataType=bfloat16  NumBuffer=1  BufferDim=[ROW,COL]  NumInput=3  NumOutput=6  RepetitionCount=0  Input0Tiling=mtxA_w(1)  Input1Tiling=mtxA_w(2)  Input2Tiling=mtxA_w(3)  Input3Tiling=[]  Input4Tiling=[]  Input5Tiling=[]  Output0Tiling=mtxA_r(1)  Output1Tiling=mtxA_r(2)  Output2Tiling=mtxA_r(3)  Output3Tiling=mtxA_r(4)  Output4Tiling=mtxA_r(5)  Output5Tiling=mtxA_r(6)  InBuffDims={256, 384}|{256, 384}|{256, 384}  InTilingDims={256, 128}|{256, 128}|{256, 128}  InOffsets={0, 0}|{0, 128}|{0, 256}  InTileTraveseDims={}|{}|{}  InTileTraveseStrides={}|{}|{}  InTileTraveseWraps={}|{}|{}  InPacketPortIDs={}|{}|{}  InRepetitions={}|{}|{}  InBoundaryDims={}|{}|{}  OutBuffDims={256, 384}|{256, 384}|{256, 384}|{256, 384}|{256, 384}|{256, 384}  OutTilingDims={256, 64}|{256, 64}|{256, 64}|{256, 64}|{256, 64}|{256, 64}  OutOffsets={0, 0}|{0, 64}|{0, 128}|{0, 192}|{0, 256}|{0, 320}  OutTileTraveseDims={}|{}|{}|{}|{}|{}  OutTileTraveseStrides={}|{}|{}|{}|{}|{}  OutTileTraveseWraps={}|{}|{}|{}|{}|{}  OutPacketPortIDs={}|{}|{}|{}|{}|{}  OutRepetitions={}|{}|{}|{}|{}|{}  OutBoundaryDims={}|{}|{}|{}|{}|{}  BufferDimStr={384, 256}  blockJsonConstraints=[]  deprecateConstraints=0
  mtxB : aieBasic/Shared Buffer  DataType=bfloat16  NumBuffer=1  BufferDim=[COL,ROW]  NumInput=6  NumOutput=3  RepetitionCount=0  Input0Tiling=mtxB_w(1)  Input1Tiling=mtxB_w(2)  Input2Tiling=mtxB_w(3)  Input3Tiling=mtxB_w(4)  Input4Tiling=mtxB_w(5)  Input5Tiling=mtxB_w(6)  Output0Tiling=mtxB_r(1)  Output1Tiling=mtxB_r(2)  Output2Tiling=mtxB_r(3)  Output3Tiling=struct('buffer_dimension', [256,384], 'tiling_dimension', [256,64], 'offset', [0,64*3])  Output4Tiling=struct('buffer_dimension', [256,384], 'tiling_dimension', [256,64], 'offset', [0,64*4])  Output5Tiling=struct('buffer_dimension', [256,384], 'tiling_dimension', [256,64], 'offset', [0,64*5])  InBuffDims={256, 384}|{256, 384}|{256, 384}|{256, 384}|{256, 384}|{256, 384}  InTilingDims={256, 64}|{256, 64}|{256, 64}|{256, 64}|{256, 64}|{256, 64}  InOffsets={0, 0}|{0, 64}|{0, 128}|{0, 192}|{0, 256}|{0, 320}  InTileTraveseDims={}|{}|{}|{}|{}|{}  InTileTraveseStrides={}|{}|{}|{}|{}|{}  InTileTraveseWraps={}|{}|{}|{}|{}|{}  InPacketPortIDs={}|{}|{}|{}|{}|{}  InRepetitions={}|{}|{}|{}|{}|{}  InBoundaryDims={}|{}|{}|{}|{}|{}  OutBuffDims={256, 384}|{256, 384}|{256, 384}  OutTilingDims={256, 128}|{256, 128}|{256, 128}  OutOffsets={0, 0}|{0, 128}|{0, 256}  OutTileTraveseDims={}|{}|{}  OutTileTraveseStrides={}|{}|{}  OutTileTraveseWraps={}|{}|{}  OutPacketPortIDs={}|{}|{}  OutRepetitions={}|{}|{}  OutBoundaryDims={}|{}|{}  BufferDimStr={256, 384}  blockJsonConstraints=[]  deprecateConstraints=0
  Out1 : Outport
  Out2 : Outport  Port=2
  Out3 : Outport  Port=3
  wires:
  PLIO5/1 -> Out3/1
  mean_dev_norm_middle3/2 -> mean_dev_norm_last/2
  PLIO2/1 -> mtxA/3
  mean_dev_norm_middle2/2 -> mean_dev_norm_middle3/3
  mtxB/3 -> PLIO5/1
  In1/1 -> PLIO/1
  PLIO3/1 -> Out1/1
  mean_dev_norm_middle/1 -> mtxB/2
  mean_dev_norm_last/1 -> mtxB/6
  PLIO4/1 -> Out2/1
  mean_dev_norm_middle1/1 -> mtxB/3
  mtxB/2 -> PLIO4/1
  mean_dev_norm_middle3/1 -> mtxB/5
  mtxB/1 -> PLIO3/1
  PLIO/1 -> mtxA/1
  PLIO1/1 -> mtxA/2
  mean_dev_norm_middle2/1 -> mtxB/4
  mean_dev_norm_middle1/2 -> mean_dev_norm_middle2/3
  mtxA/1 -> mean_dev_norm_first/1
  mean_dev_norm_first/2 -> mean_dev_norm_middle/3
  mtxA/3 -> mean_dev_norm_middle1/1
  mtxA/4 -> mean_dev_norm_middle2/1
  mtxA/5 -> mean_dev_norm_middle3/1
  mtxA/6 -> mean_dev_norm_last/1
  mean_dev_norm_last/2 -> Algebraic Loop Breaker/1
  Algebraic Loop Breaker/1 -> mean_dev_norm_first/2, mean_dev_norm_middle/2, mean_dev_norm_middle1/2, mean_dev_norm_middle2/2, mean_dev_norm_middle3/2
  In2/1 -> PLIO1/1
  In3/1 -> PLIO2/1
  mean_dev_norm_middle/2 -> mean_dev_norm_middle1/3
  mtxA/2 -> mean_dev_norm_middle/1
  mean_dev_norm_first/1 -> mtxB/1

== matlab function normalization/MATLAB Function ==
  settings: updateMethod=DISCRETE  sampleTime=1
  data: randomMatrix1 output size=ROW*COL/3; numRows parameter; numCols parameter; randomMatrix2 output size=ROW*COL/3; randomMatrix3 output size=ROW*COL/3; mean output; var output
function [randomMatrix1, randomMatrix2, randomMatrix3, mean, var] = generateRandomMatrix(numRows, numCols)

persistent p 

if isempty(p)
    p = 0;
end

randomMean = rand(1)*2^14+128;
randomGain = rand(1)*2^14+128;

if rem(p,2)==0
    randomMatrix = randn(numRows*numCols,1)*randomGain + randomMean; % Generate random matrix

    randomMatrix1 = randomMatrix(1:numRows/3*numCols);
    randomMatrix2 = randomMatrix(numRows/3*numCols+1:numRows*2/3*numCols);
    randomMatrix3 = randomMatrix(numRows*2/3*numCols+1:end);
    mean = randomMean;
    var = randomGain.^2;

else
    randomMatrix1 = [];
    randomMatrix2 = [];
    randomMatrix3 = [];
    mean = 0;
    var = 0;
end


p = p+1;
